simulink model "BevraniAGC3"  (Simulink 7.9)
settings: Solver=ode45  StartTime=0.0  StopTime=10.0  RelTol=1e-3
values from neighbouring files (symbols this model uses):
  B1 = 0.3483    [BevraniAGC3_init.m]
  B2 = 0.3827    [BevraniAGC3_init.m]
  B3 = 0.3692    [BevraniAGC3_init.m]
  D1 = 0.015    [BevraniAGC3_init.m]
  D2 = 0.016    [BevraniAGC3_init.m]
  D3 = 0.015    [BevraniAGC3_init.m]
  H1 = 0.1667/2    (= 0.08335)    [BevraniAGC3_init.m]
  H2 = 0.2017/2    (= 0.10085)    [BevraniAGC3_init.m]
  H3 = 0.1247/2    (= 0.06235)    [BevraniAGC3_init.m]
  K1 = 0.3    [BevraniAGC3_init.m]
  K2 = 0.2    [BevraniAGC3_init.m]
  K3 = 0.4    [BevraniAGC3_init.m]
  R1 = 3.00    (= 3)    [BevraniAGC3_init.m]
  R2 = 2.73    [BevraniAGC3_init.m]
  R3 = 2.82    [BevraniAGC3_init.m]
  T12 = 0.20    (= 0.2)    [BevraniAGC3_init.m]
  T13 = 0.25    [BevraniAGC3_init.m]
  T21 = 0.20    (= 0.2)    [BevraniAGC3_init.m]
  T23 = 0.12    [BevraniAGC3_init.m]
  T31 = 0.25    [BevraniAGC3_init.m]
  T32 = 0.12    [BevraniAGC3_init.m]
  Tg1 = 0.08    [BevraniAGC3_init.m]
  Tg2 = 0.06    [BevraniAGC3_init.m]
  Tg3 = 0.07    [BevraniAGC3_init.m]
  Tt1 = 0.40    (= 0.4)    [BevraniAGC3_init.m]
  Tt2 = 0.44    [BevraniAGC3_init.m]
  Tt3 = 0.30    (= 0.3)    [BevraniAGC3_init.m]
libraries: powerlib x1
settings Model: Creator=ywlaw  LastModifiedBy=ywlaw
settings GRTTargetCC: CombineOutputUpdateFcns=off  GRTInterface=on

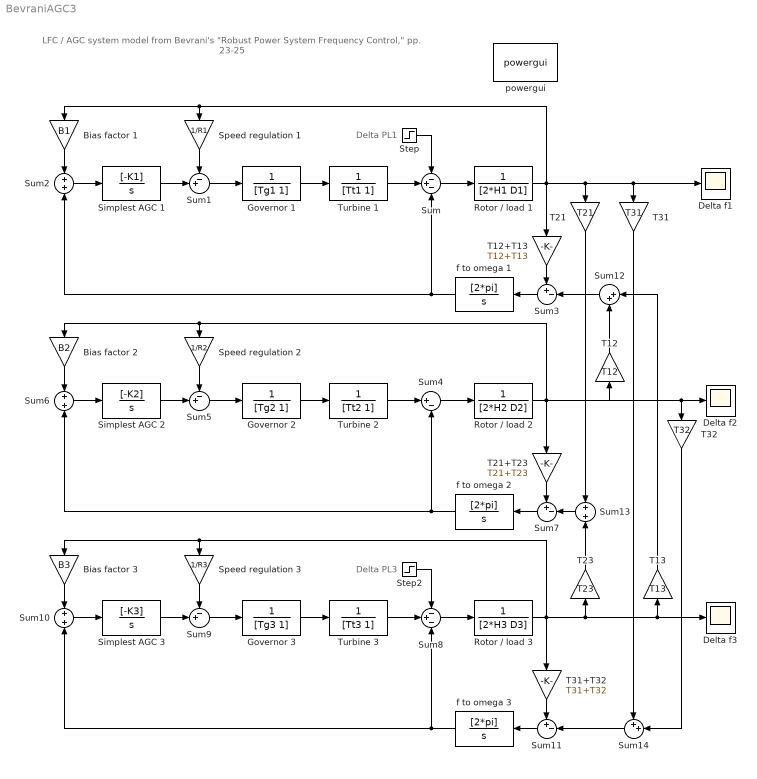
== system BevraniAGC3 ==
  note: LFC / AGC system model from Bevrani's "Robust Power System Frequency Control," pp. 23-25
  note: Delta PL1
  note: Delta PL3
  Bias factor 1 : Gain  Gain=B1
  Bias factor 2 : Gain  Gain=B2
  Bias factor 3 : Gain  Gain=B3
  Delta f1 : Scope
      settings: TimeRange=20
  Delta f2 : Scope
      settings: TimeRange=20
  Delta f3 : Scope
      settings: TimeRange=20  SaveName=ScopeData2
  Governor 1 : TransferFcn  Denominator=[Tg1 1]
  Governor 2 : TransferFcn  Denominator=[Tg2 1]
  Governor 3 : TransferFcn  Denominator=[Tg3 1]
  Rotor / load 1 : TransferFcn  Denominator=[2*H1 D1]
  Rotor / load 2 : TransferFcn  Denominator=[2*H2 D2]
  Rotor / load 3 : TransferFcn  Denominator=[2*H3 D3]
  Simplest AGC 1 : TransferFcn  Numerator=[-K1]  Denominator=[1 0]
  Simplest AGC 2 : TransferFcn  Numerator=[-K2]  Denominator=[1 0]
  Simplest AGC 3 : TransferFcn  Numerator=[-K3]  Denominator=[1 0]
  Speed regulation 1 : Gain  Gain=1/R1
  Speed regulation 2 : Gain  Gain=1/R2
  Speed regulation 3 : Gain  Gain=1/R3
  Step : Step  After=0.02  SampleTime=0  ZeroCross=off
  Step2 : Step  After=0.02  SampleTime=0  ZeroCross=off
  Sum : Sum  Inputs=-+-
  Sum1 : Sum  Inputs=-+|
  Sum{2,6,10,13} (4 alike) : Sum  Inputs=+|+
  Sum11 : Sum  Inputs=+-|
  Sum12 : Sum  Inputs=|++
  Sum14 : Sum  Inputs=++|
  Sum3 : Sum  Inputs=+-|
  Sum4 : Sum  Inputs=|+-
  Sum5 : Sum  Inputs=-+|
  Sum7 : Sum  Inputs=+-|
  Sum8 : Sum  Inputs=-+-
  Sum9 : Sum  Inputs=-+|
  T12 : Gain  Gain=T12
  T12+T13 : Gain  Gain=T12+T13
  T13 : Gain  Gain=T13
  T21 : Gain  Gain=T21
  T21+T23 : Gain  Gain=T21+T23
  T23 : Gain  Gain=T23
  T31 : Gain  Gain=T31
  T31+T32 : Gain  Gain=T31+T32
  T32 : Gain  Gain=T32
  Turbine 1 : TransferFcn  Denominator=[Tt1 1]
  Turbine 2 : TransferFcn  Denominator=[Tt2 1]
  Turbine 3 : TransferFcn  Denominator=[Tt3 1]
  f to omega 1 : TransferFcn  Numerator=[2*pi]  Denominator=[1 0]
  f to omega 2 : TransferFcn  Numerator=[2*pi]  Denominator=[1 0]
  f to omega 3 : TransferFcn  Numerator=[2*pi]  Denominator=[1 0]
  powergui : powerlib/powergui  Priority=1  SimulationMode=Continuous  SolverType=Tustin  SampleTime=50e-6  frequency=60  SPID=off  DisableSnubberDevices=off  DisableRonSwitches=off  DisableVfSwitches=off  SwTol=0  Interpol=off  DisplayEquations=off  FunctionMessages=off  frequencyindice=60  Pbase=100e6  ErrMax=1e-4  Iterations=50  UnitsV=kV  UnitsW=MW  echomessages=off  HookPort=off  EnableUseOfTLC=off  x0status=blocks  RestoreLinks=warning  ResistiveCurrentMeasurement=off  Ylog=off  Xlog=on  ShowGrid=off  save=off  variable=ZData  ZoomFFT=off  StartTime=0.0  cycles=1  DisplayStyle=1  FreqAxis=off  MaxFrequency=1000  frequencyindicesteady=1  display=off  methode=off
  wires:
  Turbine 1/1 -> Sum/2
  Governor 1/1 -> Turbine 1/1
  Sum/1 -> Rotor / load 1/1
  Sum1/1 -> Governor 1/1
  Rotor / load 1/1 -> T12+T13/1, Speed regulation 1/1, Bias factor 1/1, T21/1, Delta f1/1, T31/1
  Speed regulation 1/1 -> Sum1/1
  Simplest AGC 1/1 -> Sum1/2
  Step/1 -> Sum/1
  Sum3/1 -> f to omega 1/1
  Bias factor 1/1 -> Sum2/1
  Sum2/1 -> Simplest AGC 1/1
  f to omega 1/1 -> Sum2/2, Sum/3
  T12+T13/1 -> Sum3/1
  Governor 2/1 -> Turbine 2/1
  Sum4/1 -> Rotor / load 2/1
  Sum5/1 -> Governor 2/1
  Rotor / load 2/1 -> T12/1, T21+T23/1, Speed regulation 2/1, Bias factor 2/1, Delta f2/1, T32/1
  Speed regulation 2/1 -> Sum5/1
  Simplest AGC 2/1 -> Sum5/2
  Sum7/1 -> f to omega 2/1
  Bias factor 2/1 -> Sum6/1
  Sum6/1 -> Simplest AGC 2/1
  f to omega 2/1 -> Sum6/2, Sum4/2
  T21+T23/1 -> Sum7/1
  Turbine 3/1 -> Sum8/2
  Governor 3/1 -> Turbine 3/1
  Sum8/1 -> Rotor / load 3/1
  Sum9/1 -> Governor 3/1
  Rotor / load 3/1 -> T31+T32/1, Speed regulation 3/1, Bias factor 3/1, T23/1, Delta f3/1, T13/1
  Speed regulation 3/1 -> Sum9/1
  Simplest AGC 3/1 -> Sum9/2
  Step2/1 -> Sum8/1
  Sum11/1 -> f to omega 3/1
  Bias factor 3/1 -> Sum10/1
  Sum10/1 -> Simplest AGC 3/1
  f to omega 3/1 -> Sum10/2, Sum8/3
  T31+T32/1 -> Sum11/1
  Turbine 2/1 -> Sum4/1
  Sum12/1 -> Sum3/2
  T12/1 -> Sum12/2
  T13/1 -> Sum12/1
  Sum14/1 -> Sum11/2
  Sum13/1 -> Sum7/2
  T21/1 -> Sum13/1
  T31/1 -> Sum14/1
  T23/1 -> Sum13/2
  T32/1 -> Sum14/2
